simulink model "BESS_F_V_Controle"  (R2017b)
settings: Solver=ode45  StartTime=0.0  StopTime=10  RelTol=1e-3  EnableMultiTasking=on
values from neighbouring files (symbols this model uses):
  beta = beta (k)    [Parameter_2M_DFIG_BESS.m]
  Cbus = 80e-3    (= 0.08)    [Parameter_2M_DFIG_BESS.m]
  Cbus_bess = 15e-3    (= 0.015)    [Parameter_2M_DFIG_BESS.m]
  Cfilter = 80e-3    (= 0.08)    [Parameter_2M_DFIG_BESS.m]
  cp_opt_abs = abs(max(Cp))    [Parameter_2M_DFIG_BESS.m]
  D = 0.1    [Parameter_2M_DFIG_BESS.m]
  f = 60    [Parameter_2M_DFIG_BESS.m]
  Fs = 1.8    [Parameter_2M_DFIG_BESS.m]
  fsw = 4e3    (= 4000)    [Parameter_2M_DFIG_BESS.m]
  J = 90    [Parameter_2M_DFIG_BESS.m]
  ki_id = (wni^2)*Lr*sigma    (= 491.599501999)    [Parameter_2M_DFIG_BESS.m]
  ki_idg = (wnig^2)*Lg    (= 68.6450725305)    [Parameter_2M_DFIG_BESS.m]
  ki_iq = ki_id    (= 491.599501999)    [Parameter_2M_DFIG_BESS.m]
  ki_iqg = ki_idg    (= 68.6450725305)    [Parameter_2M_DFIG_BESS.m]
  ki_v = -300000    [Parameter_2M_DFIG_BESS.m]
  kp_id = (2*wni*sigma*Lr)-Rr    (= 0.5771)    [Parameter_2M_DFIG_BESS.m]
  kp_idg = (2*wnig*Lg)-Rg    (= 0.364153420404)    [Parameter_2M_DFIG_BESS.m]
  kp_iq = kp_id    (= 0.5771)    [Parameter_2M_DFIG_BESS.m]
  kp_iqg = kp_idg    (= 0.364153420404)    [Parameter_2M_DFIG_BESS.m]
  kp_v = -1000    [Parameter_2M_DFIG_BESS.m]
  Kpg = 1/(1.5*Vs*sqrt(2/3))    [Parameter_2M_DFIG_BESS.m]
  Kqg = -Kpg    [Parameter_2M_DFIG_BESS.m]
  lambda_opt = abs(lambda(posicion))    [Parameter_2M_DFIG_BESS.m]
  Lfilter = 483e-6    (= 0.000483)    [Parameter_2M_DFIG_BESS.m]
  Lg = 483e-6    (= 0.000483)    [Parameter_2M_DFIG_BESS.m]
  Lm = 2.5e-3    (= 0.0025)    [Parameter_2M_DFIG_BESS.m]
  Lr = Lm + Lsr    (= 0.002587)    [Parameter_2M_DFIG_BESS.m]
  Ls = Lm + Lsi    (= 0.002587)    [Parameter_2M_DFIG_BESS.m]
  Lsi = 87e-6    (= 8.7e-05)    [Parameter_2M_DFIG_BESS.m]
  N = 100    [Parameter_2M_DFIG_BESS.m]
  p = 2    [Parameter_2M_DFIG_BESS.m]
  Ps = 2e6    (= 2000000)    [Parameter_2M_DFIG_BESS.m]
  Radio = 44    [Parameter_2M_DFIG_BESS.m]
  Rfilter = 20e-3    (= 0.02)    [Parameter_2M_DFIG_BESS.m]
  Rg = 20e-6    (= 2e-05)    [Parameter_2M_DFIG_BESS.m]
  ro = 1.225    [Parameter_2M_DFIG_BESS.m]
  Rr = 2.9e-3    (= 0.0029)    [Parameter_2M_DFIG_BESS.m]
  Rs = 2.6e-3    (= 0.0026)    [Parameter_2M_DFIG_BESS.m]
  sigma = 1- Lm^2/(Ls*Lr)    (= 0.0661284179513)    [Parameter_2M_DFIG_BESS.m]
  Ts = 1/fsw/f    (= 4.16666666667e-06)    [Parameter_2M_DFIG_BESS.m]
  Vbus_ref = 1200    [Parameter_2M_DFIG_BESS.m]
  Vdc_bat_ref = 1300    [Parameter_2M_DFIG_BESS.m]
  Vs = 690    [Parameter_2M_DFIG_BESS.m]
undefined symbols (not defined in the file or in its folder): D1, D11, Delta, DiscIntNeverNeededParam, Ion, Lithium, sigbuilder_block
libraries: powerlib x61, powerlib_meascontrol x31, electricdrivelib x1, sps_avr x1
(part 1 of 3)
settings Model: SimulationMode=accelerator  Creator=admin  LastModifiedBy=admin
settings DataIOCC: LimitDataPoints=on  SaveFormat=Array
settings OptimizationCC: EfficientMapNaN2IntZero=off  LifeSpan=inf
settings DebuggingCC: UnderspecifiedInitializationDetection=Classic  MergeDetectMultiDrivingBlocksExec=none  SolverPrmCheckMsg=warning  StateNameClashWarn=warning  SFUnexpectedBacktrackingDiag=warning  SFNoUnconditionalDefaultTransitionDiag=warning  SFExecutionAtInitializationDiag=none
settings HardwareCC: ProdBitPerPointer=32  ProdBitPerSizeT=32  ProdBitPerPtrDiffT=32  ProdLargestAtomicFloat=None  ProdIntDivRoundTo=Undefined  ProdEndianess=Unspecified  ProdWordSize=32  ProdHWDeviceType=32-bit Generic  TargetBitPerPointer=64  TargetBitPerSizeT=64  TargetBitPerPtrDiffT=64  TargetLongLongMode=on  TargetIntDivRoundTo=Zero  TargetEndianess=LittleEndian  TargetWordSize=64  TargetHWDeviceType=MATLAB Host  ProdEqTarget=off
settings ModelReferenceCC: PropagateSignalLabelsOutOfModel=off
settings CodeAppCC: MaxIdLength=128
settings GRTTargetCC: TargetLangStandard=C89/C90 (ANSI)  CombineOutputUpdateFcns=off  GRTInterface=on
settings ConfigComp: CovMetricSettings=dw  CovHtmlReporting=on  CovSaveCumulativeToWorkspaceVar=on  CovSaveSingleToWorkspaceVar=on  CovExternalEMLEnable=off
settings SimscapeCC: SimscapeNormalizeSystem=off

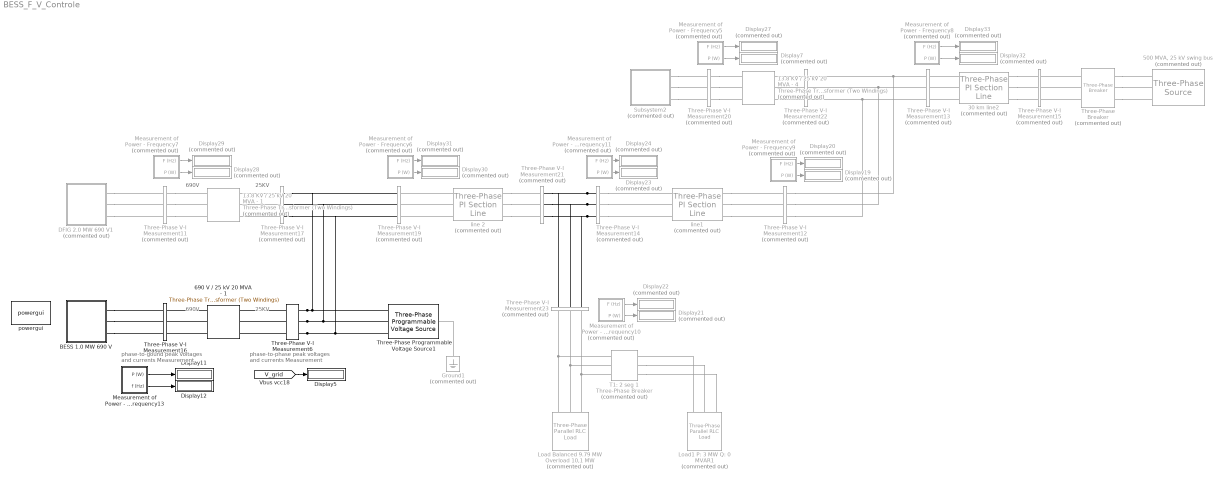
== system BESS_F_V_Controle ==
  note: 25KV
  note: 690V
  note: 690V
  note: 25KV
  note: phase-to-phase peak voltages
      | and currents Measurement
  note: phase-to-gound peak voltages
      | and currents Measurement
  " line 2 " : powerlib/Elements/Three-Phase PI Section Line  Commented=on  LConnTagsString=a|b|c  RConnTagsString=A|B|C  Frequency=f  Resistances=[0.1153 0.413]  Inductances=[1.05e-3 3.32e-3]  Capacitances=[11.33e-009 5.01e-009]  Length=1
      settings: SourceProductName=Simscape Power Systems
  " line1" : powerlib/Elements/Three-Phase PI Section Line  Commented=on  LConnTagsString=a|b|c  RConnTagsString=A|B|C  Frequency=f  Resistances=[0.1153 0.413]  Inductances=[1.05e-3 3.32e-3]  Capacitances=[11.33e-009 5.01e-009]  Length=15
      settings: SourceProductName=Simscape Power Systems
  13.8 KV / 25 kV 20 MVA - 1 : powerlib/Elements/Three-Phase Transformer (Two Windings)  Commented=on  Winding1Connection=Delta (D11)  Winding2Connection=Yg  CoreType=Three single-phase transformers  SetSaturation=off  Hysteresis=off  DataFile='hysteresis'  SetInitialFlux=off  Measurements=None  UNITS=SI  NominalPower=[20e6 f]  Winding1=[25000 0.14881 0.011842]  Winding2=[690 2.624e-05 2.0881e-06]  Rm=89286  Lm=Inf  L0=0.5  Saturation=[0 0;0.47518 112.54;197.99 142.55]  InitialFluxes=[75.026 -75.026 65.648]  MoreParameters=off  BreakLoop=off  DataType=on  TransfoNumber=0
  13.8 KV / 25 kV 20 MVA - 4 : powerlib/Elements/Three-Phase Transformer (Two Windings)  Commented=on  Winding1Connection=Delta (D11)  Winding2Connection=Yg  CoreType=Three single-phase transformers  SetSaturation=off  Hysteresis=off  DataFile='hysteresis'  SetInitialFlux=off  Measurements=None  UNITS=SI  NominalPower=[20e6 f]  Winding1=[25000 0.14881 0.011842]  Winding2=[13800 2.624e-05 2.0881e-06]  Rm=89286  Lm=Inf  L0=0.5  Saturation=[0 0;0.47518 112.54;197.99 142.55]  InitialFluxes=[75.026 -75.026 65.648]  MoreParameters=off  BreakLoop=off  DataType=on  TransfoNumber=0
  30 km line2 : powerlib/Elements/Three-Phase PI Section Line  Commented=on  LConnTagsString=a|b|c  RConnTagsString=A|B|C  Frequency=f  Resistances=[0.1153 0.413]  Inductances=[1.05e-3 3.32e-3]  Capacitances=[11.33e-009 5.01e-009]  Length=3
      settings: SourceProductName=Simscape Power Systems
  "500 MVA, 25 kV swing bus" : powerlib/Electrical Sources/Three-Phase Source  Commented=on  InternalConnection=Yg  VoltagePhases=off  Voltage=25e3  PhaseAngle=0  Voltage_phases=[25e3 25e3 25e3]/sqrt(3)  PhaseAngles_phases=[0 -120 +120]  Frequency=f  NonIdealSource=on  SpecifyImpedance=on  Resistance=0  Inductance=47.147e-3  ShortCircuitLevel=500e6  BaseVoltage=25e3  XRratio=100  BusType=swing  Pref=10e3  Qref=0  Prefabc=[10e3, 10e3, 10e3]  Qrefabc=[0, 0, 0]  Qmin=-inf  Qmax=inf
  690 V / 25 kV 20 MVA - 1 : powerlib/Elements/Three-Phase Transformer (Two Windings)  Winding1Connection=Delta (D11)  Winding2Connection=Yg  CoreType=Three single-phase transformers  SetSaturation=off  Hysteresis=off  DataFile='hysteresis'  SetInitialFlux=off  Measurements=None  UNITS=SI  NominalPower="[20e6  f]"  Winding1=[25000 0.14881 0.011842]  Winding2=[690 200e-3 2.0881e-06]  Rm=89286  Lm=Inf  L0=0.5  Saturation=[0 0;0.47518 112.54;197.99 142.55]  InitialFluxes=[75.026 -75.026 65.648]  MoreParameters=off  BreakLoop=off  DataType=on  TransfoNumber=0
  BESS 1.0 MW 690 V : Subsystem
  DFIG 2.0 MW 690 V1 : Subsystem  Commented=on
  Display11 : Display
  Display12 : Display
  Display{7,19..24,27..33} (14 alike) : Display  Commented=on
  Display5 : Display
  Ground1 : powerlib/Elements/Ground  Commented=on  LConnTagsString=a
  "Load Balanced 9.79 MW Overload 10,1 MW " : powerlib/Elements/Three-Phase Parallel RLC Load  Commented=on  LConnTagsString=A|B|C  Configuration=Y (grounded)  NominalVoltage=25e3  Vabc=[1e3 1e3 1e3]  Vabcp=[1e3 1e3 1e3]  NominalFrequency=f  UnbalancedPower=off  ActivePower=9.79e6  InductivePower=0  CapacitivePower=0  Pabc=[10e3 9e3 11e3]  QLabc=[100 90 110]  QCabc=[100 90 110]  Pabcp=[10e3 9e3 11e3]  QLabcp=[100 90 110]  QCabcp=[100 90 110]  Measurements=None  LoadType=constant I
  Load1 P: 3 MW Q: 0 MVAR1 : powerlib/Elements/Three-Phase Parallel RLC Load  Commented=on  LConnTagsString=A|B|C  Configuration=Y (grounded)  NominalVoltage=25e3  Vabc=[1e3 1e3 1e3]  Vabcp=[1e3 1e3 1e3]  NominalFrequency=f  UnbalancedPower=off  ActivePower=3e6  InductivePower=0  CapacitivePower=0  Pabc=[10e3 9e3 11e3]  QLabc=[100 90 110]  QCabc=[100 90 110]  Pabcp=[10e3 9e3 11e3]  QLabcp=[100 90 110]  QCabcp=[100 90 110]  Measurements=None  LoadType=constant I
  Measurement of Power - Frequency10 : Subsystem  Commented=on
  Measurement of Power - Frequency11 : Subsystem  Commented=on
  Measurement of Power - Frequency13 : Subsystem
  Measurement of Power - Frequency5 : Subsystem  Commented=on
  Measurement of Power - Frequency6 : Subsystem  Commented=on
  Measurement of Power - Frequency7 : Subsystem  Commented=on
  Measurement of Power - Frequency8 : Subsystem  Commented=on
  Measurement of Power - Frequency9 : Subsystem  Commented=on
  Subsystem2 : Subsystem  Commented=on
  T1: 2 seg 1 : powerlib/Elements/Three-Phase Breaker  Commented=on  InitialState=open  SwitchA=on  SwitchB=on  SwitchC=on  SwitchTimes=2  External=off  BreakerResistance=0.01  SnubberResistance=5e6  SnubberCapacitance=inf  Measurements=None
  Three-Phase Programmable Voltage Source1 : powerlib/Electrical Sources/Three-Phase Programmable Voltage Source  PositiveSequence="[25e3  0 f]"  VariationEntity=Amplitude  VariationType=Table of time-amplitude pairs  VariationTypeAlt=Step  VariationStep=-0.8  VariationRate=10  VariationMagnitude=0.3  VariationFrequency=2  VariationTiming=[0.5 3]  VariationPhaseA=off  Amplitudes=[1 0.95 1]  TimeValues=[0 0.9 2]  HarmonicGeneration=off  HarmonicA=[3 0.2 -25 0]  HarmonicB=[2 0.15 35 2]  Timing="[0.05  3]"  BusType=swing  Pref=0  Qref=0  Qmin=-inf  Qmax=inf
  Three-Phase V-I Measurement11 : powerlib/Measurements/Three-Phase V-I Measurement  Commented=on  VoltageMeasurement=phase-to-ground  SetLabelV=on  LabelV=V_ac_dfig_low  Vpu=off  VpuLL=off  CurrentMeasurement=yes  SetLabelI=on  LabelI=I_ac_dfig_low  Ipu=off  Pbase=100e6  Vbase=500e3  OutputType=Complex  PhasorSimulation=off  PSBequivalent=0
  Three-Phase V-I Measurement12 : powerlib/Measurements/Three-Phase V-I Measurement  Commented=on  VoltageMeasurement=phase-to-ground  SetLabelV=on  LabelV=V_ac_line_4  Vpu=off  VpuLL=off  CurrentMeasurement=yes  SetLabelI=on  LabelI=I_ac_line_4  Ipu=off  Pbase=100e6  Vbase=500e3  OutputType=Complex  PhasorSimulation=off  PSBequivalent=0
  Three-Phase V-I Measurement13 : powerlib/Measurements/Three-Phase V-I Measurement  Commented=on  VoltageMeasurement=phase-to-ground  SetLabelV=on  LabelV=V_ac_syn_slack  Vpu=off  VpuLL=off  CurrentMeasurement=yes  SetLabelI=on  LabelI=I_ac_syn_slack  Ipu=off  Pbase=100e6  Vbase=500e3  OutputType=Complex  PhasorSimulation=off  PSBequivalent=0
  Three-Phase V-I Measurement14 : powerlib/Measurements/Three-Phase V-I Measurement  Commented=on  VoltageMeasurement=phase-to-ground  SetLabelV=on  LabelV=V_ac_line_3  Vpu=off  VpuLL=off  CurrentMeasurement=yes  SetLabelI=on  LabelI=I_ac_line_3  Ipu=off  Pbase=100e6  Vbase=500e3  OutputType=Complex  PhasorSimulation=off  PSBequivalent=0
  Three-Phase V-I Measurement15 : powerlib/Measurements/Three-Phase V-I Measurement  Commented=on  VoltageMeasurement=phase-to-ground  SetLabelV=on  LabelV=V_ac_syn_slack2  Vpu=off  VpuLL=off  CurrentMeasurement=yes  SetLabelI=on  LabelI=I_ac_syn_slack2  Ipu=off  Pbase=100e6  Vbase=500e3  OutputType=Complex  PhasorSimulation=off  PSBequivalent=0
  Three-Phase V-I Measurement16 : powerlib/Measurements/Three-Phase V-I Measurement  VoltageMeasurement=phase-to-phase  SetLabelV=on  LabelV=V_ac_bat_low  Vpu=off  VpuLL=off  CurrentMeasurement=yes  SetLabelI=on  LabelI=I_ac_bat_low  Ipu=off  Pbase=100e6  Vbase=500e3  OutputType=Complex  PhasorSimulation=off  PSBequivalent=0
  Three-Phase V-I Measurement17 : powerlib/Measurements/Three-Phase V-I Measurement  Commented=on  VoltageMeasurement=phase-to-phase  SetLabelV=on  LabelV=V_ac_dfig_H  Vpu=off  VpuLL=off  CurrentMeasurement=yes  SetLabelI=on  LabelI=I_ac_dfig_H  Ipu=off  Pbase=100e6  Vbase=500e3  OutputType=Complex  PhasorSimulation=off  PSBequivalent=0
  Three-Phase V-I Measurement19 : powerlib/Measurements/Three-Phase V-I Measurement  Commented=on  VoltageMeasurement=phase-to-ground  SetLabelV=on  LabelV=V_ac_line_1  Vpu=off  VpuLL=off  CurrentMeasurement=yes  SetLabelI=on  LabelI=I_ac_line_1  Ipu=off  Pbase=100e6  Vbase=500e3  OutputType=Complex  PhasorSimulation=off  PSBequivalent=0
  Three-Phase V-I Measurement20 : powerlib/Measurements/Three-Phase V-I Measurement  Commented=on  VoltageMeasurement=phase-to-ground  SetLabelV=on  LabelV=V_ac_syn_low  Vpu=off  VpuLL=off  CurrentMeasurement=yes  SetLabelI=on  LabelI=I_ac_syn_low  Ipu=off  Pbase=100e6  Vbase=500e3  OutputType=Complex  PhasorSimulation=off  PSBequivalent=0
  Three-Phase V-I Measurement21 : powerlib/Measurements/Three-Phase V-I Measurement  Commented=on  VoltageMeasurement=phase-to-ground  SetLabelV=on  LabelV=V_ac_line_2  Vpu=off  VpuLL=off  CurrentMeasurement=yes  SetLabelI=on  LabelI=I_ac_line_2  Ipu=off  Pbase=100e6  Vbase=500e3  OutputType=Complex  PhasorSimulation=off  PSBequivalent=0
  Three-Phase V-I Measurement22 : powerlib/Measurements/Three-Phase V-I Measurement  Commented=on  VoltageMeasurement=phase-to-ground  SetLabelV=on  LabelV=V_ac_syn_H  Vpu=off  VpuLL=off  CurrentMeasurement=yes  SetLabelI=on  LabelI=I_ac_syn_H  Ipu=off  Pbase=100e6  Vbase=500e3  OutputType=Complex  PhasorSimulation=off  PSBequivalent=0
  Three-Phase V-I Measurement23 : powerlib/Measurements/Three-Phase V-I Measurement  Commented=on  VoltageMeasurement=phase-to-ground  SetLabelV=on  LabelV=V_ac_load  Vpu=off  VpuLL=off  CurrentMeasurement=yes  SetLabelI=on  LabelI=I_ac_load  Ipu=off  Pbase=100e6  Vbase=500e3  OutputType=Complex  PhasorSimulation=off  PSBequivalent=0
  Three-Phase V-I Measurement6 : powerlib/Measurements/Three-Phase V-I Measurement  VoltageMeasurement=phase-to-phase  SetLabelV=on  LabelV=V_ac_g  Vpu=off  VpuLL=off  CurrentMeasurement=yes  SetLabelI=on  LabelI=I_ac_g  Ipu=off  Pbase=100e6  Vbase=500e3  OutputType=Complex  PhasorSimulation=off  PSBequivalent=0
  Three-Phase Breaker : powerlib/Elements/Three-Phase Breaker  Commented=on  InitialState=closed  SwitchA=on  SwitchB=on  SwitchC=on  SwitchTimes=2.5  External=off  BreakerResistance=0.01  SnubberResistance=1e6  SnubberCapacitance=inf  Measurements=None
  powergui : powerlib/powergui  Priority=1  SimulationMode=Discrete  SampleTime=Ts  frequency=60  Iterations=50  frequencyindice=60  Pbase=100e6  ErrMax=1e-4  UnitsV=kV  UnitsW=MW  buscounter=0  FunctionMessages=off  echomessages=off  EnableUseOfTLC=off  CurrentSourceSwitches=off  DisableSnubberDevices=off  DisableRonSwitches=off  DisableVfSwitches=off  DisplayEquations=off  SolverType=Tustin  Interpol=off  ExternalGateDelay=off  methode=off  Ts=0  x0status=blocks  SPID=off  SwTol=0  HookPort=off  RestoreLinks=warning  ResistiveCurrentMeasurement=off  Frange=[0:2:500]  Ylog=off  Xlog=on  ShowGrid=off  save=off  variable=ZData  structure=0  ZoomFFT=off  StartTime=0.0  cycles=1  DisplayStyle=1  fundamental=60  FreqAxis=off  MaxFrequency=1000  frequencyindicesteady=1  RmsSteady=1  display=off
  wires:
  Measurement of Power - Frequency11/1(F (Hz)) -> Display24/1
  Measurement of Power - Frequency8/2(P (W)) -> Display32/1
  Measurement of Power - Frequency8/1(F (Hz)) -> Display33/1
  Measurement of Power - Frequency10/1(F (Hz)) -> Display22/1
  Measurement of Power - Frequency9/1(F (Hz)) -> Display20/1
  Measurement of Power - Frequency9/2(P (W)) -> Display19/1
  Measurement of Power - Frequency7/1(F (Hz)) -> Display29/1
  Measurement of Power - Frequency5/1(F (Hz)) -> Display27/1
  Measurement of Power - Frequency7/2(P (W)) -> Display28/1
  Measurement of Power - Frequency6/1(F (Hz)) -> Display31/1
  Measurement of Power - Frequency6/2(P (W)) -> Display30/1
  Measurement of Power - Frequency10/2(P (W)) -> Display21/1
  Measurement of Power - Frequency11/2(P (W)) -> Display23/1
  Measurement of Power - Frequency5/2(P (W)) -> Display7/1
  Measurement of Power - Frequency13/2(f (Hz)) -> Display12/1
  Measurement of Power - Frequency13/1(P (W)) -> Display11/1
  [V_grid] -> Display5/1
  connections:
  Three-Phase V-I Measurement13/LConn1 -- Three-Phase V-I Measurement12/RConn1 -- Three-Phase V-I Measurement22/RConn1
  Three-Phase V-I Measurement13/LConn3 -- Three-Phase V-I Measurement12/RConn3 -- Three-Phase V-I Measurement22/RConn3
  Three-Phase V-I Measurement14/LConn3 -- Three-Phase V-I Measurement21/RConn3 -- Three-Phase V-I Measurement23/LConn1
  Three-Phase V-I Measurement14/LConn2 -- Three-Phase V-I Measurement21/RConn2 -- Three-Phase V-I Measurement23/LConn2
  Three-Phase V-I Measurement13/LConn2 -- Three-Phase V-I Measurement12/RConn2 -- Three-Phase V-I Measurement22/RConn2
  Three-Phase V-I Measurement14/LConn1 -- Three-Phase V-I Measurement21/RConn1 -- Three-Phase V-I Measurement23/LConn3
  Three-Phase V-I Measurement6/LConn1 -- 690 V / 25 kV 20 MVA - 1/LConn1
  " line1"/RConn2 -- Three-Phase V-I Measurement12/LConn2
  "Load Balanced 9.79 MW Overload 10,1 MW "/LConn3 -- T1: 2 seg 1/LConn3 -- Three-Phase V-I Measurement23/RConn1
  13.8 KV / 25 kV 20 MVA - 1/LConn1 -- Three-Phase V-I Measurement17/LConn1
  " line 2 "/LConn1 -- Three-Phase V-I Measurement19/RConn1
  BESS 1.0 MW 690 V/RConn3 -- Three-Phase V-I Measurement16/LConn3
  Three-Phase V-I Measurement11/RConn1 -- 13.8 KV / 25 kV 20 MVA - 1/RConn1
  690 V / 25 kV 20 MVA - 1/RConn3 -- Three-Phase V-I Measurement16/RConn3
  Subsystem2/LConn1 -- Three-Phase V-I Measurement20/LConn1
  Three-Phase V-I Measurement11/RConn2 -- 13.8 KV / 25 kV 20 MVA - 1/RConn2
  Three-Phase V-I Measurement6/LConn2 -- 690 V / 25 kV 20 MVA - 1/LConn2
  13.8 KV / 25 kV 20 MVA - 1/LConn3 -- Three-Phase V-I Measurement17/LConn3
  30 km line2/RConn3 -- Three-Phase V-I Measurement15/LConn3
  13.8 KV / 25 kV 20 MVA - 1/LConn2 -- Three-Phase V-I Measurement17/LConn2
  Three-Phase V-I Measurement14/RConn3 -- " line1"/LConn3
  30 km line2/LConn1 -- Three-Phase V-I Measurement13/RConn1
  690 V / 25 kV 20 MVA - 1/RConn2 -- Three-Phase V-I Measurement16/RConn2
  Three-Phase V-I Measurement14/RConn1 -- " line1"/LConn1
  690 V / 25 kV 20 MVA - 1/RConn1 -- Three-Phase V-I Measurement16/RConn1
  DFIG 2.0 MW 690 V1/RConn1 -- Three-Phase V-I Measurement11/LConn1
  Three-Phase V-I Measurement20/RConn2 -- 13.8 KV / 25 kV 20 MVA - 4/RConn2
  Three-Phase V-I Measurement14/RConn2 -- " line1"/LConn2
  Subsystem2/LConn3 -- Three-Phase V-I Measurement20/LConn3
  Three-Phase V-I Measurement6/LConn3 -- 690 V / 25 kV 20 MVA - 1/LConn3
  30 km line2/RConn1 -- Three-Phase V-I Measurement15/LConn1
  "Load Balanced 9.79 MW Overload 10,1 MW "/LConn2 -- T1: 2 seg 1/LConn2 -- Three-Phase V-I Measurement23/RConn2
  Three-Phase V-I Measurement22/LConn1 -- 13.8 KV / 25 kV 20 MVA - 4/LConn1
  DFIG 2.0 MW 690 V1/RConn3 -- Three-Phase V-I Measurement11/LConn3
  30 km line2/RConn2 -- Three-Phase V-I Measurement15/LConn2
  Three-Phase V-I Measurement20/RConn3 -- 13.8 KV / 25 kV 20 MVA - 4/RConn3
  30 km line2/LConn2 -- Three-Phase V-I Measurement13/RConn2
  Three-Phase V-I Measurement22/LConn3 -- 13.8 KV / 25 kV 20 MVA - 4/LConn3
  DFIG 2.0 MW 690 V1/RConn2 -- Three-Phase V-I Measurement11/LConn2
  " line 2 "/RConn2 -- Three-Phase V-I Measurement21/LConn2
  "Load Balanced 9.79 MW Overload 10,1 MW "/LConn1 -- T1: 2 seg 1/LConn1 -- Three-Phase V-I Measurement23/RConn3
  " line 2 "/LConn3 -- Three-Phase V-I Measurement19/RConn3
  " line 2 "/LConn2 -- Three-Phase V-I Measurement19/RConn2
  " line 2 "/RConn3 -- Three-Phase V-I Measurement21/LConn3
  BESS 1.0 MW 690 V/RConn1 -- Three-Phase V-I Measurement16/LConn1
  Three-Phase V-I Measurement22/LConn2 -- 13.8 KV / 25 kV 20 MVA - 4/LConn2
  " line 2 "/RConn1 -- Three-Phase V-I Measurement21/LConn1
  " line1"/RConn1 -- Three-Phase V-I Measurement12/LConn1
  " line1"/RConn3 -- Three-Phase V-I Measurement12/LConn3
  Three-Phase V-I Measurement11/RConn3 -- 13.8 KV / 25 kV 20 MVA - 1/RConn3
  Subsystem2/LConn2 -- Three-Phase V-I Measurement20/LConn2
  30 km line2/LConn3 -- Three-Phase V-I Measurement13/RConn3
  Three-Phase V-I Measurement20/RConn1 -- 13.8 KV / 25 kV 20 MVA - 4/RConn1
  BESS 1.0 MW 690 V/RConn2 -- Three-Phase V-I Measurement16/LConn2
  Three-Phase V-I Measurement6/RConn3 -- Three-Phase Programmable Voltage Source1/RConn3 -- Three-Phase V-I Measurement19/LConn3 -- Three-Phase V-I Measurement17/RConn3
  Three-Phase V-I Measurement6/RConn2 -- Three-Phase Programmable Voltage Source1/RConn2 -- Three-Phase V-I Measurement19/LConn2 -- Three-Phase V-I Measurement17/RConn2
  Three-Phase V-I Measurement6/RConn1 -- Three-Phase Programmable Voltage Source1/RConn1 -- Three-Phase V-I Measurement17/RConn1 -- Three-Phase V-I Measurement19/LConn1
  Ground1/LConn1 -- Three-Phase Programmable Voltage Source1/LConn1
  T1: 2 seg 1/RConn2 -- Load1 P: 3 MW Q: 0 MVAR1/LConn2
  T1: 2 seg 1/RConn3 -- Load1 P: 3 MW Q: 0 MVAR1/LConn3
  Load1 P: 3 MW Q: 0 MVAR1/LConn1 -- T1: 2 seg 1/RConn1
  Three-Phase Breaker/RConn1 -- "500 MVA, 25 kV swing bus"/RConn1
  Three-Phase Breaker/RConn2 -- "500 MVA, 25 kV swing bus"/RConn2
  Three-Phase Breaker/RConn3 -- "500 MVA, 25 kV swing bus"/RConn3
  Three-Phase Breaker/LConn1 -- Three-Phase V-I Measurement15/RConn1
  Three-Phase Breaker/LConn2 -- Three-Phase V-I Measurement15/RConn2
  Three-Phase Breaker/LConn3 -- Three-Phase V-I Measurement15/RConn3

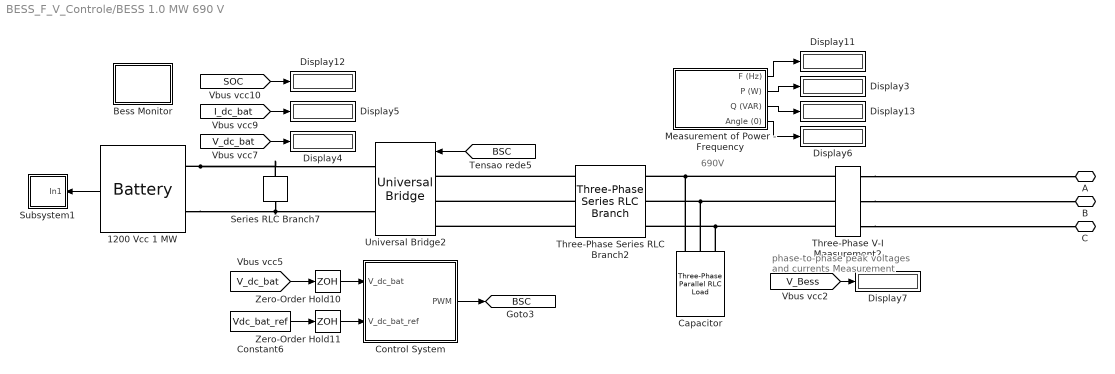
== system BESS_F_V_Controle/BESS 1.0 MW 690 V ==
  note: 690V
  note: phase-to-phase peak voltages
      | and currents Measurement
  "1200 Vcc 1 MW " : electricdrivelib/Extra Sources/Battery  BatType=Lithium-Ion  ShowTempParam=off  ThermalPreset=no  ShowAgeParam=off  NomV=1200  NomQ=833  SOC=71  Batt_Tr=30  PresetModel=on  MaxQ=833  MinV=900  FullV=1396.7846  Dis_rate=362.1739  R=0.014406  Normal_OP=753.3217  expZone="[1296.463      40.925652]"  current=[833]  Units=Time  Tci=20  NomT=25  T2=0  MaxQ2=2.208  FullV2=3.45  Normal_OP2=2.8  expZone2="[3.22        0.23]"  Rca=0.6  ti=1000  Dp=0  Neq0=0  Tsim=1e6  Ta1=25  Qeol=5.4*0.9  Reol=0.013333*1.2  Char_age=[2.3478, 3]  Dis_age=[2.3478, 10]  N1=1500  N2=10500  N3=1000  N4=1400  Ta2=45  N5=950
  Bess Monitor : Subsystem
  Capacitor : powerlib/Elements/Three-Phase Parallel RLC Load  LConnTagsString=A|B|C  Configuration=Y (grounded)  NominalVoltage=Vs  Vabc=[1e3 1e3 1e3]  Vabcp=[1e3 1e3 1e3]  NominalFrequency=f  UnbalancedPower=off  ActivePower=0  InductivePower=0  CapacitivePower=Cfilter*2.5  Pabc=[10e3 9e3 11e3]  QLabc=[100 90 110]  QCabc=[100 90 110]  Pabcp=[10e3 9e3 11e3]  QLabcp=[100 90 110]  QCabcp=[100 90 110]  Measurements=None  LoadType=constant Z
  Constant6 : Constant  Value=Vdc_bat_ref
  Control System : Subsystem
  Display{3..7,11..13} (8 alike) : Display
  Measurement of Power - Frequency : Subsystem
  Series RLC Branch7 : powerlib/Elements/Series RLC Branch  LConnTagsString=__new0  RConnTagsString=__new0  BranchType=C  Resistance=1  Inductance=1e-3  SetiL0=off  InitialCurrent=0  Capacitance=Cbus_bess  Setx0=off  InitialVoltage=0  Measurements=Branch voltage
  Subsystem1 : Subsystem
  Three-Phase Series RLC Branch2 : powerlib/Elements/Three-Phase Series RLC Branch  LConnTagsString=A|B|C  RConnTagsString=A|B|C  BranchType=RL  Resistance=Rfilter  Inductance=Lfilter*1.5  Capacitance=0  Measurements=None
  Three-Phase V-I Measurement2 : powerlib/Measurements/Three-Phase V-I Measurement  VoltageMeasurement=phase-to-phase  SetLabelV=on  LabelV=V_ac_bess  Vpu=off  VpuLL=off  CurrentMeasurement=yes  SetLabelI=on  LabelI=I_ac_bess  Ipu=off  Pbase=100e6  Vbase=Vs  OutputType=Complex  PhasorSimulation=off  PSBequivalent=0
  Universal Bridge2 : powerlib/Power Electronics/Universal Bridge  Arms=3  SnubberResistance=1e5  SnubberCapacitance=inf  Device=Ideal Switches  Ron=1e-3  Lon=0  ForwardVoltages="[  0  0  ]"  ForwardVoltage=0  GTOparameters=[ 10e-6 , 20e-6 ]  IGBTparameters=[ 1e-6 , 2e-6 ]  Measurements=None  Measurements_2=None  converterType=Rectifier
  Zero-Order Hold10 : ZeroOrderHold  SampleTime=1/fsw
  Zero-Order Hold11 : ZeroOrderHold  SampleTime=1/fsw
  A : PMIOPort  Port=1  Side=Right
  B : PMIOPort  Port=2  Side=Right
  C : PMIOPort  Port=3  Side=Right
  tag scope: BSC=global
  wires:
  Zero-Order Hold10/1 -> Control System/1(V_dc_bat)
  [V_dc_bat] -> Zero-Order Hold10/1
  [I_dc_bat] -> Display5/1
  Control System/1(PWM) -> [BSC]
  Zero-Order Hold11/1 -> Control System/2(V_dc_bat_ref)
  [V_dc_bat] -> Display4/1
  "1200 Vcc 1 MW "/1 -> Subsystem1/1(In1)
  Constant6/1 -> Zero-Order Hold11/1
  [BSC] -> Universal Bridge2/1
  Measurement of Power - Frequency/2(P (W)) -> Display3/1
  Measurement of Power - Frequency/1(F (Hz)) -> Display11/1
  Measurement of Power - Frequency/3(Q (VAR)) -> Display13/1
  [SOC] -> Display12/1
  Measurement of Power - Frequency/4(Angle (0)) -> Display6/1
  [V_Bess] -> Display7/1
  connections:
  Series RLC Branch7/RConn1 -- "1200 Vcc 1 MW "/LConn2 -- Universal Bridge2/RConn2
  "1200 Vcc 1 MW "/LConn1 -- Series RLC Branch7/LConn1 -- Universal Bridge2/RConn1
  Capacitor/LConn1 -- Three-Phase V-I Measurement2/LConn1 -- Three-Phase Series RLC Branch2/RConn1
  Capacitor/LConn2 -- Three-Phase V-I Measurement2/LConn2 -- Three-Phase Series RLC Branch2/RConn2
  Capacitor/LConn3 -- Three-Phase V-I Measurement2/LConn3 -- Three-Phase Series RLC Branch2/RConn3
  Three-Phase Series RLC Branch2/LConn1 -- Universal Bridge2/LConn1
  Three-Phase Series RLC Branch2/LConn2 -- Universal Bridge2/LConn2
  Three-Phase Series RLC Branch2/LConn3 -- Universal Bridge2/LConn3
  Three-Phase V-I Measurement2/RConn1 -- A/RConn1
  Three-Phase V-I Measurement2/RConn2 -- B/RConn1
  Three-Phase V-I Measurement2/RConn3 -- C/RConn1

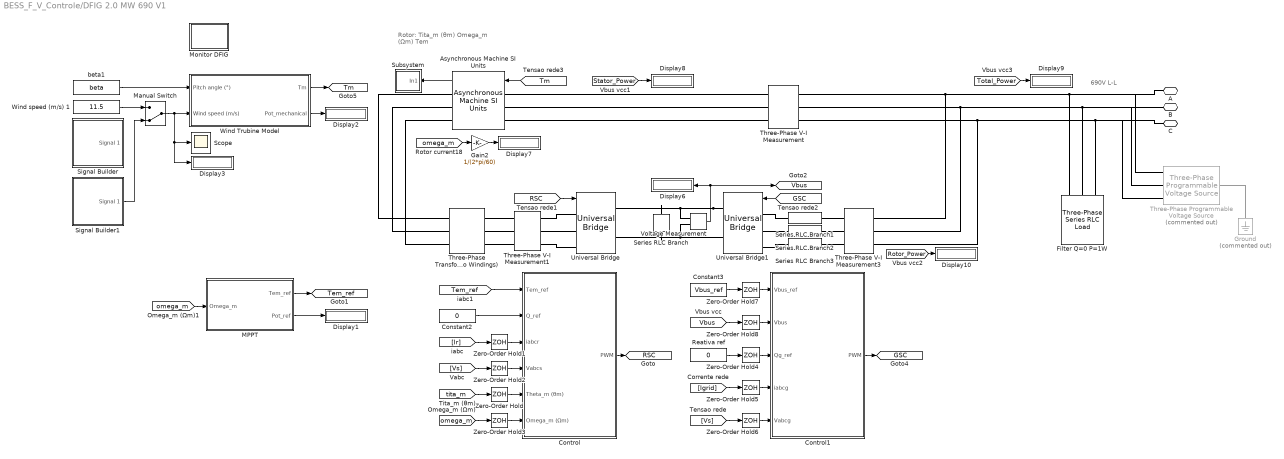
== system BESS_F_V_Controle/DFIG 2.0 MW 690 V1 ==
  note: 690V L-L
  note: Rotor:
      | Tita_m (θm)
      | Omega_m (Ωm)
      | Tem
  Asynchronous Machine SI Units : powerlib/Machines/Asynchronous Machine SI Units  RotorType=Wound  PresetModel=No  MechanicalLoad=Torque Tm  ShowDetailedParameters=on  ReferenceFrame=Rotor  Units=SI  MeasurementBus=off  NominalParameters=[ Ps Vs f ]  Stator=[ Rs , Lsi]  Rotor=[ Rr , Lsi]  Cage1=[ 0.022 0.226/377]  Cage2=[ 0.022 0.226/377]  Lm=Lm  Mechanical=[ J D 2 ]  PolePairs=2  InitialConditions=[1 0 0 0 0 0 0 0]  SimulateSaturation=off  Saturation=[14.03593122, 27.81365428, 53.79336849, 72.68890987, 97.98006896, 148.6815601, 215.7428561, 302.9841135, 420.4778367 ; 230, 322, 414, 460, 506, 552, 598, 644, 690]  LoadFlowParameters=1492000  TsPowergui=0  TsBlock=-1  IterativeModel=Trapezoidal non iterative  IterativeDiscreteModel=Trapezoidal non iterative  Pmec=0
  Constant2 : Constant  Value=0
  Constant3 : Constant  Value=Vbus_ref
  Control : Subsystem
  Control1 : Subsystem
  Display{1..3,6..10} (8 alike) : Display
  Filter Q=0 P=1W : powerlib/Elements/Three-Phase Series RLC Load  LConnTagsString=A|B|C  Configuration=Y (grounded)  NominalVoltage=Vs  Vabc=[1e3 1e3 1e3]  Vabcp=[1e3 1e3 1e3]  NominalFrequency=f  UnbalancedPower=off  ActivePower=1  InductivePower=0  CapacitivePower=0  Pabc=[10e3 9e3 11e3]  QLabc=[100 90 110]  QCabc=[100 90 110]  Pabcp=[10e3 9e3 11e3]  QLabcp=[100 90 110]  QCabcp=[100 90 110]  Measurements=None  LoadType=constant Z
  Gain2 : Gain  Gain=1/(2*pi/60)
  Ground : powerlib/Elements/Ground  Commented=on  LConnTagsString=a
  MPPT : Subsystem
  Manual Switch : ManualSwitch  CurrentSetting=0
  Monitor DFIG : Subsystem
  Reativa ref : Constant  Value=0
  Scope : Scope
  Series RLC Branch : powerlib/Elements/Series RLC Branch  LConnTagsString=__new0  RConnTagsString=__new0  BranchType=C  Resistance=1  Inductance=1e-3  SetiL0=off  InitialCurrent=0  Capacitance=Cbus  Setx0=off  InitialVoltage=0  Measurements=Branch voltage
  Series RLC Branch1 : powerlib/Elements/Series RLC Branch  LConnTagsString=__new0  RConnTagsString=__new0  BranchType=RL  Resistance=Rg  Inductance=Lg  SetiL0=off  InitialCurrent=0  Capacitance=0  Setx0=off  InitialVoltage=0  Measurements=None
  Series RLC Branch2 : powerlib/Elements/Series RLC Branch  LConnTagsString=__new0  RConnTagsString=__new0  BranchType=RL  Resistance=Rg  Inductance=Lg  SetiL0=off  InitialCurrent=0  Capacitance=0  Setx0=off  InitialVoltage=0  Measurements=None
  Series RLC Branch3 : powerlib/Elements/Series RLC Branch  LConnTagsString=__new0  RConnTagsString=__new0  BranchType=RL  Resistance=Rg  Inductance=Lg  SetiL0=off  InitialCurrent=0  Capacitance=0  Setx0=off  InitialVoltage=0  Measurements=None
  Signal Builder : Subsystem  Tag=STV Subsys  LoadFcn=sigbuilder_block('load');  StartFcn=sigbuilder_block('start');  StopFcn=sigbuilder_block('stop');  ClipboardFcn=sigbuilder_block('clipboard');  mask(Sigbuilder block){tuvar=[0:10]}
      mask help: Simulink:masks:SigbuilderBlock_MD
      mask init:
      | if ~strcmp(get_param(bdroot(gcbh),'SimulationStatus'),'stopped') tuvar = sigbuilder_block('maskInit'); end
      settings: CopyFcn=sigbuilder_block('copy');  DeleteFcn=sigbuilder_block('delete');  ModelCloseFcn=sigbuilder_block('modelClose');  PreSaveFcn=sigbuilder_block('preSave');  PauseFcn=sigbuilder_block('pause');  ContinueFcn=sigbuilder_block('continue');  NameChangeFcn=sigbuilder_block('namechange');  OpenFcn=sigbuilder_block('open',[6 22.5 1012.5 455.25 ]);  CloseFcn=sigbuilder_block('close');
      mask Display: plot(0, 0, 100, 100,[2, 2, 32, 32, 2], [68, 8, 8, 68, 68],[32, 2], [38, 38], [32, 19, 2],[53, 60, 44], [32, 17, 17, 2],[16, 16, 31, 31]);txt = getActiveGroup(gcbh);text(2, 100, txt,'verticalAlignment', 'top');
  Signal Builder1 : Subsystem  Tag=STV Subsys  LoadFcn=sigbuilder_block('load');  StartFcn=sigbuilder_block('start');  StopFcn=sigbuilder_block('stop');  ClipboardFcn=sigbuilder_block('clipboard');  mask(Sigbuilder block){tuvar=[0:10]}
      mask help: Simulink:masks:SigbuilderBlock_MD
      mask init:
      | if ~strcmp(get_param(bdroot(gcbh),'SimulationStatus'),'stopped') tuvar = sigbuilder_block('maskInit'); end
      settings: CopyFcn=sigbuilder_block('copy');  DeleteFcn=sigbuilder_block('delete');  ModelCloseFcn=sigbuilder_block('modelClose');  PreSaveFcn=sigbuilder_block('preSave');  PauseFcn=sigbuilder_block('pause');  ContinueFcn=sigbuilder_block('continue');  NameChangeFcn=sigbuilder_block('namechange');  OpenFcn=sigbuilder_block('open',[0 22.5 1024.5 495.75 ]);  CloseFcn=sigbuilder_block('close');
      mask Display: plot(0, 0, 100, 100,[2, 2, 32, 32, 2], [68, 8, 8, 68, 68],[32, 2], [38, 38], [32, 19, 2],[53, 60, 44], [32, 17, 17, 2],[16, 16, 31, 31]);txt = getActiveGroup(gcbh);text(2, 100, txt,'verticalAlignment', 'top');
  Subsystem : Subsystem
  Three-Phase Programmable Voltage Source : powerlib/Electrical Sources/Three-Phase Programmable Voltage Source  Commented=on  PositiveSequence="[Vs  0 f]"  VariationEntity=Frequency  VariationType=Table of time-amplitude pairs  VariationTypeAlt=Step  VariationStep=-0.8  VariationRate=10  VariationMagnitude=0.3  VariationFrequency=2  VariationTiming=[0.2 3]  VariationPhaseA=off  Amplitudes=[1 0.8 1.2 1.0]  TimeValues=[0 0.1 0.15 0.2]  HarmonicGeneration=off  HarmonicA=[3 0.2 -25 0]  HarmonicB=[2 0.15 35 2]  Timing="[0.05  3]"  BusType=swing  Pref=0  Qref=0  Qmin=-inf  Qmax=inf
  Three-Phase Transformer (Two Windings) : powerlib/Elements/Three-Phase Transformer (Two Windings)  Winding1Connection=Y  Winding2Connection=Y  CoreType=Three single-phase transformers  SetSaturation=off  Hysteresis=off  DataFile='hysteresis'  SetInitialFlux=off  Measurements=None  UNITS=SI  NominalPower=[ Ps , f]  Winding1=[Vs 0 0]  Winding2=[Vs/u 0 0]  Rm=1.0805e+06  Lm=2866  L0=0.5  Saturation=[0 0;0.66653 1910.3;277.72 2419.7]  InitialFluxes=[1273.5 -1273.5 1114.3]  MoreParameters=off  BreakLoop=off  DataType=on  TransfoNumber=1
  Three-Phase V-I Measurement : powerlib/Measurements/Three-Phase V-I Measurement  VoltageMeasurement=phase-to-ground  SetLabelV=on  LabelV=Vs  Vpu=off  VpuLL=off  CurrentMeasurement=yes  SetLabelI=on  LabelI=Is  Ipu=off  Pbase=100e6  Vbase=500e3  OutputType=Complex  PhasorSimulation=off  PSBequivalent=0
  Three-Phase V-I Measurement1 : powerlib/Measurements/Three-Phase V-I Measurement  VoltageMeasurement=phase-to-phase  SetLabelV=on  LabelV=Vr  Vpu=off  VpuLL=off  CurrentMeasurement=yes  SetLabelI=on  LabelI=Ir  Ipu=off  Pbase=100e6  Vbase=500e3  OutputType=Complex  PhasorSimulation=off  PSBequivalent=0
  Three-Phase V-I Measurement3 : powerlib/Measurements/Three-Phase V-I Measurement  VoltageMeasurement=phase-to-ground  SetLabelV=on  LabelV=Vgrid  Vpu=off  VpuLL=off  CurrentMeasurement=yes  SetLabelI=on  LabelI=Igrid  Ipu=off  Pbase=100e6  Vbase=500e3  OutputType=Complex  PhasorSimulation=off  PSBequivalent=0
  Universal Bridge : powerlib/Power Electronics/Universal Bridge  Arms=3  SnubberResistance=1e5  SnubberCapacitance=inf  Device=Ideal Switches  Ron=1e-3  Lon=0  ForwardVoltages="[  0  0  ]"  ForwardVoltage=0  GTOparameters=[ 10e-6 , 20e-6 ]  IGBTparameters=[ 1e-6 , 2e-6 ]  Measurements=None  Measurements_2=None  converterType=Rectifier
  Universal Bridge1 : powerlib/Power Electronics/Universal Bridge  Arms=3  SnubberResistance=1e5  SnubberCapacitance=inf  Device=Ideal Switches  Ron=1e-3  Lon=0  ForwardVoltages="[  0  0  ]"  ForwardVoltage=0  GTOparameters=[ 10e-6 , 20e-6 ]  IGBTparameters=[ 1e-6 , 2e-6 ]  Measurements=None  Measurements_2=None  converterType=Rectifier
  Voltage Measurement : powerlib/Measurements/Voltage Measurement  PhasorSimulation=off  OutputType=Complex  PSBequivalent=0
  Wind Trubine Model : Subsystem
  Wind speed (m/s) 1 : Constant  Value=11.5
  Zero-Order Hold{,1..8} (9 alike) : ZeroOrderHold  SampleTime=1/fsw
  beta1 : Constant  Value=beta
  A : PMIOPort  Port=1  Side=Right
  B : PMIOPort  Port=2  Side=Right
  C : PMIOPort  Port=3  Side=Right
  tag scope: GSC=global, RSC=global, Tem_ref=global, Tm=global, Vbus=global
  wires:
  [Igrid] -> Zero-Order Hold5/1
  beta1/1 -> Wind Trubine Model/1(Pitch angle (°))
  Constant3/1 -> Zero-Order Hold7/1
  MPPT/1(Tem_ref) -> [Tem_ref]
  Wind Trubine Model/1(Tm) -> [Tm]
  [Stator_Power] -> Display8/1
  [Tm] -> Asynchronous Machine SI Units/1
  MPPT/2("Pot_ref ") -> Display1/1
  Reativa ref/1 -> Zero-Order Hold4/1
  [GSC] -> Universal Bridge1/1
  Wind Trubine Model/2(Pot_mechanical) -> Display2/1
  [omega_m] -> MPPT/1(Omega_m)
  Control/1(PWM) -> [RSC]
  [tita_m] -> Zero-Order Hold/1
  [Tem_ref] -> Control/1(Tem_ref)
  [Rotor_Power] -> Display10/1
  [omega_m] -> Gain2/1
  [Vs] -> Zero-Order Hold2/1
  Asynchronous Machine SI Units/1 -> Subsystem/1(In1)
  Zero-Order Hold/1 -> Control/5(Theta_m (θm))
  Zero-Order Hold2/1 -> Control/4(Vabcs)
  [omega_m] -> Zero-Order Hold3/1
  Gain2/1 -> Display7/1
  Zero-Order Hold1/1 -> Control/3(iabcr)
  Constant2/1 -> Control/2(Q_ref)
  [Vbus] -> Zero-Order Hold8/1
  Zero-Order Hold7/1 -> Control1/1(Vbus_ref)
  [RSC] -> Universal Bridge/1
  Zero-Order Hold3/1 -> Control/6("Omega_m (Ωm) ")
  [Ir] -> Zero-Order Hold1/1
  [Vs] -> Zero-Order Hold6/1
  [Total_Power] -> Display9/1
  Zero-Order Hold6/1 -> Control1/5("Vabcg ")
  Zero-Order Hold5/1 -> Control1/4(iabcg)
  Voltage Measurement/1 -> Display6/1, [Vbus]
  Zero-Order Hold4/1 -> Control1/3(Qg_ref)
  Control1/1(PWM) -> [GSC]
  Zero-Order Hold8/1 -> Control1/2(Vbus)
  Manual Switch/1 -> Display3/1, Scope/1, Wind Trubine Model/2(Wind speed (m/s))
  Wind speed (m/s) 1/1 -> Manual Switch/1
  Signal Builder1/1(Signal 1) -> Manual Switch/2
  connections:
  Three-Phase V-I Measurement/RConn2 -- Three-Phase Programmable Voltage Source/RConn2 -- B/RConn1 -- Filter Q=0 P=1W/LConn2 -- Three-Phase V-I Measurement3/RConn2
  Three-Phase V-I Measurement/RConn1 -- Three-Phase Programmable Voltage Source/RConn1 -- A/RConn1 -- Filter Q=0 P=1W/LConn1 -- Three-Phase V-I Measurement3/RConn1
  Voltage Measurement/LConn2 -- Universal Bridge1/RConn2 -- Universal Bridge/RConn2 -- Series RLC Branch/RConn1
  Universal Bridge1/RConn1 -- Voltage Measurement/LConn1 -- Universal Bridge/RConn1 -- Series RLC Branch/LConn1
  Three-Phase V-I Measurement/RConn3 -- Three-Phase Programmable Voltage Source/RConn3 -- C/RConn1 -- Filter Q=0 P=1W/LConn3 -- Three-Phase V-I Measurement3/RConn3
  Three-Phase Transformer (Two Windings)/LConn2 -- Asynchronous Machine SI Units/RConn2
  Three-Phase Transformer (Two Windings)/LConn3 -- Asynchronous Machine SI Units/RConn3
  Three-Phase V-I Measurement3/LConn2 -- Series RLC Branch2/RConn1
  Three-Phase V-I Measurement1/LConn1 -- Universal Bridge/LConn1
  Three-Phase V-I Measurement/LConn1 -- Asynchronous Machine SI Units/LConn1
  Three-Phase V-I Measurement3/LConn3 -- Series RLC Branch3/RConn1
  Three-Phase Transformer (Two Windings)/LConn1 -- Asynchronous Machine SI Units/RConn1
  Three-Phase V-I Measurement/LConn3 -- Asynchronous Machine SI Units/LConn3
  Three-Phase V-I Measurement3/LConn1 -- Series RLC Branch1/RConn1
  Three-Phase Transformer (Two Windings)/RConn3 -- Three-Phase V-I Measurement1/RConn3
  Three-Phase V-I Measurement1/LConn3 -- Universal Bridge/LConn3
  Universal Bridge1/LConn1 -- Series RLC Branch1/LConn1
  Three-Phase V-I Measurement1/LConn2 -- Universal Bridge/LConn2
  Three-Phase Transformer (Two Windings)/RConn2 -- Three-Phase V-I Measurement1/RConn2
  Universal Bridge1/LConn3 -- Series RLC Branch3/LConn1
  Three-Phase V-I Measurement/LConn2 -- Asynchronous Machine SI Units/LConn2
  Universal Bridge1/LConn2 -- Series RLC Branch2/LConn1
  Three-Phase Transformer (Two Windings)/RConn1 -- Three-Phase V-I Measurement1/RConn1
  Ground/LConn1 -- Three-Phase Programmable Voltage Source/LConn1

== system BESS_F_V_Controle/Measurement of Power - Frequency10 ==
  PLL (3ph)1 : powerlib_meascontrol/PLL/PLL (3ph)  Commented=on  Fmin=45  Par_Init=[0, f]  ParK=[180, 3200, 1]  TcD=1e-4  MaxRateChangeFreq=12  FilterCutOffFreq=25  Ts=0  AGC=on
  "Power (3ph, Instantaneous)1" : powerlib_meascontrol/Measurements/Power (3ph, Instantaneous)
      settings: SourceProductName=Simscape Power Systems
  F (Hz) : Outport
  P (W) : Outport  Port=2
  wires:
  [I_ac_load] -> "Power (3ph, Instantaneous)1"/2
  PLL (3ph)1/1 -> F (Hz)/1
  "Power (3ph, Instantaneous)1"/1 -> P (W)/1  "Pot"
  [V_ac_load] -> PLL (3ph)1/1, "Power (3ph, Instantaneous)1"/1

== system BESS_F_V_Controle/Measurement of Power - Frequency11 ==
  PLL (3ph)1 : powerlib_meascontrol/PLL/PLL (3ph)  Commented=on  Fmin=45  Par_Init=[0, f]  ParK=[180, 3200, 1]  TcD=1e-4  MaxRateChangeFreq=12  FilterCutOffFreq=25  Ts=0  AGC=on
  "Power (3ph, Instantaneous)1" : powerlib_meascontrol/Measurements/Power (3ph, Instantaneous)
      settings: SourceProductName=Simscape Power Systems
  F (Hz) : Outport
  P (W) : Outport  Port=2
  wires:
  [I_ac_line_3] -> "Power (3ph, Instantaneous)1"/2
  PLL (3ph)1/1 -> F (Hz)/1
  "Power (3ph, Instantaneous)1"/1 -> P (W)/1  "Pot"
  [V_ac_line_3] -> PLL (3ph)1/1, "Power (3ph, Instantaneous)1"/1

== system BESS_F_V_Controle/Measurement of Power - Frequency13 ==
  PLL (3ph)1 : powerlib_meascontrol/PLL/PLL (3ph)  Fmin=45  Par_Init=[0, f]  ParK=[180, 3200, 1]  TcD=1e-4  MaxRateChangeFreq=12  FilterCutOffFreq=25  Ts=0  AGC=on
  "Power (3ph, Instantaneous)1" : powerlib_meascontrol/Measurements/Power (3ph, Instantaneous)
      settings: SourceProductName=Simscape Power Systems
  P (W) : Outport
  f (Hz) : Outport  Port=2
  tag scope: f_g=global
  wires:
  [V_ac_bat_low] -> PLL (3ph)1/1, "Power (3ph, Instantaneous)1"/1
  "Power (3ph, Instantaneous)1"/1 -> P (W)/1  "Pot"
  [I_ac_bat_low] -> "Power (3ph, Instantaneous)1"/2
  PLL (3ph)1/1 -> [f_g], f (Hz)/1

== system BESS_F_V_Controle/Measurement of Power - Frequency5 ==
  PLL (3ph)1 : powerlib_meascontrol/PLL/PLL (3ph)  Commented=on  Fmin=45  Par_Init=[0, f]  ParK=[180, 3200, 1]  TcD=1e-4  MaxRateChangeFreq=12  FilterCutOffFreq=25  Ts=0  AGC=on
  "Power (3ph, Instantaneous)1" : powerlib_meascontrol/Measurements/Power (3ph, Instantaneous)
      settings: SourceProductName=Simscape Power Systems
  F (Hz) : Outport
  P (W) : Outport  Port=2
  wires:
  [I_ac_syn_low] -> "Power (3ph, Instantaneous)1"/2
  PLL (3ph)1/1 -> F (Hz)/1
  "Power (3ph, Instantaneous)1"/1 -> P (W)/1  "Pot"
  [V_ac_syn_low] -> PLL (3ph)1/1, "Power (3ph, Instantaneous)1"/1

== system BESS_F_V_Controle/Measurement of Power - Frequency6 ==
  PLL (3ph)1 : powerlib_meascontrol/PLL/PLL (3ph)  Commented=on  Fmin=45  Par_Init=[0, f]  ParK=[180, 3200, 1]  TcD=1e-4  MaxRateChangeFreq=12  FilterCutOffFreq=25  Ts=0  AGC=on
  "Power (3ph, Instantaneous)1" : powerlib_meascontrol/Measurements/Power (3ph, Instantaneous)
      settings: SourceProductName=Simscape Power Systems
  F (Hz) : Outport
  P (W) : Outport  Port=2
  wires:
  [I_ac_line_1] -> "Power (3ph, Instantaneous)1"/2
  PLL (3ph)1/1 -> F (Hz)/1
  "Power (3ph, Instantaneous)1"/1 -> P (W)/1  "Pot"
  [V_ac_line_1] -> PLL (3ph)1/1, "Power (3ph, Instantaneous)1"/1

== system BESS_F_V_Controle/Measurement of Power - Frequency7 ==
  PLL (3ph)1 : powerlib_meascontrol/PLL/PLL (3ph)  Commented=on  Fmin=45  Par_Init=[0, f]  ParK=[180, 3200, 1]  TcD=1e-4  MaxRateChangeFreq=12  FilterCutOffFreq=25  Ts=0  AGC=on
  "Power (3ph, Instantaneous)1" : powerlib_meascontrol/Measurements/Power (3ph, Instantaneous)
      settings: SourceProductName=Simscape Power Systems
  F (Hz) : Outport
  P (W) : Outport  Port=2
  wires:
  [I_ac_dfig_low] -> "Power (3ph, Instantaneous)1"/2
  PLL (3ph)1/1 -> F (Hz)/1
  "Power (3ph, Instantaneous)1"/1 -> P (W)/1  "Pot"
  [V_ac_dfig_low] -> PLL (3ph)1/1, "Power (3ph, Instantaneous)1"/1

== system BESS_F_V_Controle/Measurement of Power - Frequency8 ==
  PLL (3ph)1 : powerlib_meascontrol/PLL/PLL (3ph)  Fmin=45  Par_Init=[0, f]  ParK=[180, 3200, 1]  TcD=1e-4  MaxRateChangeFreq=12  FilterCutOffFreq=25  Ts=0  AGC=on
  "Power (3ph, Instantaneous)1" : powerlib_meascontrol/Measurements/Power (3ph, Instantaneous)
      settings: SourceProductName=Simscape Power Systems
  F (Hz) : Outport
  P (W) : Outport  Port=2
  wires:
  [V_ac_syn_slack] -> "Power (3ph, Instantaneous)1"/1, PLL (3ph)1/1
  "Power (3ph, Instantaneous)1"/1 -> P (W)/1  "Pot"
  PLL (3ph)1/1 -> F (Hz)/1
  [I_ac_syn_slack] -> "Power (3ph, Instantaneous)1"/2

== system BESS_F_V_Controle/Measurement of Power - Frequency9 ==
  PLL (3ph)1 : powerlib_meascontrol/PLL/PLL (3ph)  Commented=on  Fmin=45  Par_Init=[0, f]  ParK=[180, 3200, 1]  TcD=1e-4  MaxRateChangeFreq=12  FilterCutOffFreq=25  Ts=0  AGC=on
  "Power (3ph, Instantaneous)1" : powerlib_meascontrol/Measurements/Power (3ph, Instantaneous)
      settings: SourceProductName=Simscape Power Systems
  F (Hz) : Outport
  P (W) : Outport  Port=2
  wires:
  [V_ac_line_4] -> "Power (3ph, Instantaneous)1"/1, PLL (3ph)1/1
  "Power (3ph, Instantaneous)1"/1 -> P (W)/1  "Pot"
  PLL (3ph)1/1 -> F (Hz)/1
  [I_ac_line_4] -> "Power (3ph, Instantaneous)1"/2
